simulink model "code_gen_man_bin"  (Simulink 7.5)
settings: Solver=FixedStepDiscrete  SolverMode=SingleTasking  StartTime=0.0  StopTime=10.0  FixedStep=0.01  RelTol=1e-3
InitFcn:
  | boat_constants
values from neighbouring files (symbols this model uses):
  figure8_waypoints = int32([ ... (first row only)    [boat_constants.m]
  InitialPoint = 0    [boat_constants.m]    (also in l2plus.m)
  IPStar = 0    [boat_constants.m]    (also in l2plus.m)
  ISA_g = 9.815    [boat_constants.m]
  MaxDwnPthStar = 1    [boat_constants.m]    (also in l2plus.m)
  OC2max = 49999    [boat_constants.m]    (also in simulation_constants.m)
  sampling_waypoints = int32([ ... (first row only)    [boat_constants.m]
  switchDistance = 4    [boat_constants.m]    (also in l2plus.m)
  T_step = 0.01    [boat_constants.m]    (also in common.m)
  tanIntercept = tan( 45*pi/180 )    [boat_constants.m]    (also in l2plus.m)
  test_waypoints = int32([ ... (first row only)    [boat_constants.m]
  TStar = single(4.5)    [boat_constants.m]    (also in l2plus.m = single(2))
  Turn2Track = 0    [boat_constants.m]    (also in l2plus.m)
  wheelbase = 3.27    [boat_constants.m]
undefined symbols (not defined in the file or in its folder): clearGpsData, clearSensorData, cpInitCommunications, DataEEInitAndClear, DataEEWrite, DiscIntNeverNeededParam, ecan1_buffered_transmit_matlab, ecan1_error_status_matlab, ecan1_init, GetAirData, getGpsData, getRevoData, getSensorData, GetThrottleData, GetWaterData, GetWindData, Init_onlyOnce, Init_Reset, initCalibrationRange, initGps, processNewCommData, processNewGpsData, processNewRevoData, setHilMode, u1, u2, uart1EnqueueStateData, uart2EnqueueActuatorData, y1
libraries: simulink x80, dsPICdrivers x50, uSimLib x4, simulink_need_slupdate x4
(part 4 of 6)

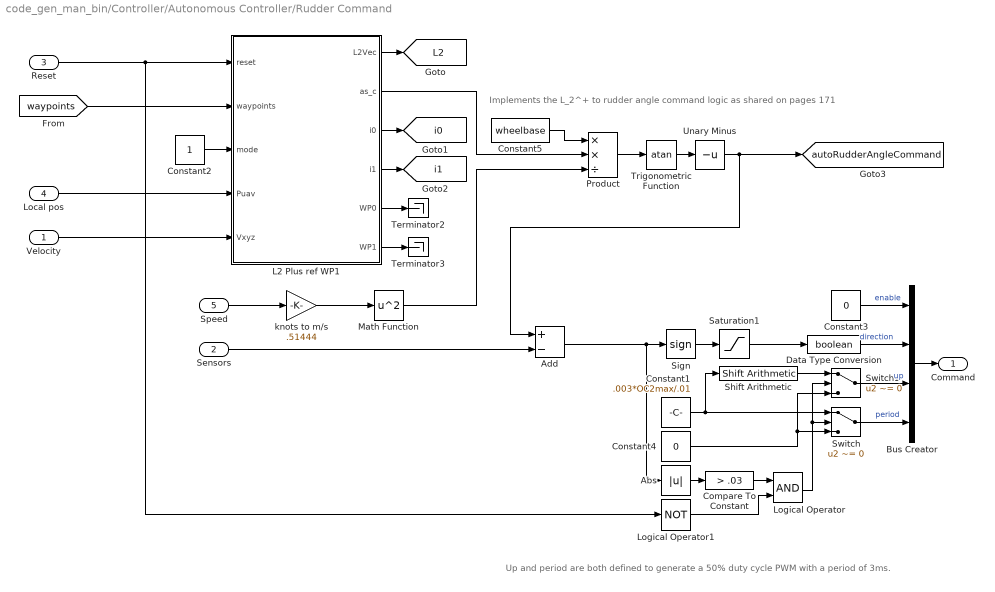
== system code_gen_man_bin/Controller/Autonomous Controller/Rudder Command ==
  note: Implements the L_2^+ to rudder angle command logic as shared on pages 171
  note: Up and period are both defined to generate a 50% duty cycle PWM with
      | a period of 3ms.
  Velocity : Inport
  Sensors : Inport  Port=2
  Reset : Inport  Port=3
  Local pos : Inport  Port=4
  Speed : Inport  Port=5
  Abs : Abs  OutDataType=fixdt(1, 16)  OutScaling=2^0
  Add : Sum  Inputs=+-  OutDataType=fixdt(1, 16)  OutScaling=2^-10
  Bus Creator : BusCreator
  Compare To Constant : simulink/Logic and Bit Operations/Compare To Constant  SystemSampleTime=-1  relop=>  const=.03  LogicOutDataTypeMode=boolean
  Constant1 : Constant  Value=.003*OC2max/.01  OutDataTypeMode=uint16  OutDataType=sfix(16)  OutScaling=2^0  OutDataTypeStr=uint16
  Constant2 : Constant  OutDataTypeMode=uint8  OutDataType=sfix(16)  OutScaling=2^0  OutDataTypeStr=uint8
  Constant3 : Constant  Value=0  OutDataTypeMode=boolean  OutDataType=sfix(16)  OutScaling=2^0  OutDataTypeStr=boolean
  Constant4 : Constant  Value=0  OutDataTypeMode=uint16  OutDataType=sfix(16)  OutScaling=2^0  OutDataTypeStr=uint16
  Constant5 : Constant  Value=wheelbase  OutDataTypeMode=boolean  OutDataType=sfix(16)  OutScaling=2^0  OutDataTypeStr=boolean
  Data Type Conversion : DataTypeConversion  OutDataTypeMode=boolean  OutDataType=fixdt(1, 16)  OutScaling=2^0  OutDataTypeStr=boolean  RndMeth=Simplest
  L2 Plus ref WP1 : Stateflow chart  TreatAsAtomicUnit=on
  Logical Operator : Logic  AllPortsSameDT=off  OutDataTypeMode=boolean  LogicDataType=fixdt(0, 8)  OutDataTypeStr=boolean
  Logical Operator1 : Logic  Operator=NOT  Inputs=1  AllPortsSameDT=off  OutDataTypeMode=boolean  LogicDataType=fixdt(0, 8)  OutDataTypeStr=boolean
  Math Function : Math  Operator=square  OutDataType=fixdt(1, 16)  OutScaling=2^0  SaturateOnIntegerOverflow=on
  Product : Product  Inputs=**/  OutDataType=fixdt(1, 16)  OutScaling=2^0  RndMeth=Zero
  Saturation1 : Saturate  UpperLimit=1  LowerLimit=0  OutDataTypeStr=Inherit: Inherit via back propagation
  Shift Arithmetic : simulink/Logic and Bit Operations/Shift Arithmetic  SystemSampleTime=-1  nBitShiftRight=1  nBinPtShiftRight=0
  Sign : Signum
  Switch : Switch  Criteria=u2 ~= 0  OutDataType=fixdt(1, 16)  OutScaling=2^0
  Switch1 : Switch  Criteria=u2 ~= 0  OutDataType=fixdt(1, 16)  OutScaling=2^0
  Terminator2 : Terminator
  Terminator3 : Terminator
  Trigonometric Function : Trigonometry  Operator=atan
  Unary Minus : UnaryMinus
  knots to m/s : Gain  Gain=.51444  ParameterDataType=fixdt(1, 16)  ParameterScaling=2^0  OutDataType=fixdt(1, 16)  OutScaling=2^0
  Command : Outport
  tag scope: L2=global, autoRudderAngleCommand=global, i0=global, i1=global
  wires:
  Unary Minus/1 -> [autoRudderAngleCommand], Add/1
  knots to m/s/1 -> Math Function/1
  Trigonometric Function/1 -> Unary Minus/1
  Product/1 -> Trigonometric Function/1
  Math Function/1 -> Product/3
  Constant5/1 -> Product/1
  L2 Plus ref WP1/6(WP1) -> Terminator3/1
  L2 Plus ref WP1/5(WP0) -> Terminator2/1
  L2 Plus ref WP1/2(as_c) -> Product/2
  Data Type Conversion/1 -> Bus Creator/2  "direction"
  Sensors/1 -> Add/2
  Bus Creator/1 -> Command/1
  Saturation1/1 -> Data Type Conversion/1
  Sign/1 -> Saturation1/1
  Constant2/1 -> L2 Plus ref WP1/3(mode)
  L2 Plus ref WP1/1(L2Vec) -> [L2]
  Velocity/1 -> L2 Plus ref WP1/5(Vxyz)
  Constant3/1 -> Bus Creator/1  "enable"
  Constant1/1 -> Shift Arithmetic/1, Switch/1
  Abs/1 -> Compare To Constant/1
  Shift Arithmetic/1 -> Switch1/1
  Switch/1 -> Bus Creator/4  "period"
  Switch1/1 -> Bus Creator/3  "up"
  Constant4/1 -> Switch/3, Switch1/3
  Reset/1 -> L2 Plus ref WP1/1(reset), Logical Operator1/1
  Local pos/1 -> L2 Plus ref WP1/4(Puav)
  L2 Plus ref WP1/3(i0) -> [i0]
  L2 Plus ref WP1/4(i1) -> [i1]
  Compare To Constant/1 -> Logical Operator/1
  Logical Operator/1 -> Switch/2, Switch1/2
  Logical Operator1/1 -> Logical Operator/2
  [waypoints] -> L2 Plus ref WP1/2(waypoints)
  Speed/1 -> knots to m/s/1
  Add/1 -> Sign/1, Abs/1

== system code_gen_man_bin/Controller/Autonomous Controller/State Keeper & Estimator ==
  throttle : Inport
  rudder : Inport  Port=2
  reset : Inport  Port=3
  gps : Inport  Port=4
  ballast : Inport  Port=5
  Ballast Estimator : Subsystem
  GPS Estimator : Subsystem
  Rudder Estimator : Subsystem
  Throttle Estimator : Subsystem
  sensors_t : Outport
  sensors_r : Outport  Port=2
  sensors_b : Outport  Port=3
  velocity : Outport  Port=4
  pos : Outport  Port=5
  heading : Outport  Port=6
  lla : Outport  Port=7
  datetime : Outport  Port=8
  tag scope: SensedGlobalPosition=global, SensedHeading=global, SensedLocalPosition=global, SensedVelocity=global
  wires:
  rudder/1 -> Rudder Estimator/1(r)
  ballast/1 -> Ballast Estimator/1(b)
  throttle/1 -> Throttle Estimator/1(t)
  reset/1 -> GPS Estimator/2(reset)
  GPS Estimator/1(velocity) -> velocity/1, [SensedVelocity]
  gps/1 -> GPS Estimator/1(gps)
  GPS Estimator/2(pos) -> pos/1, [SensedLocalPosition]
  GPS Estimator/3(heading) -> heading/1, [SensedHeading]
  GPS Estimator/4(lla) -> [SensedGlobalPosition], lla/1
  GPS Estimator/5(datetime) -> datetime/1
  Rudder Estimator/1(sensors_r) -> sensors_r/1
  Ballast Estimator/1(sensors_b) -> sensors_b/1
  Throttle Estimator/1(sensors_t) -> sensors_t/1

== system code_gen_man_bin/Controller/Autonomous Controller/Throttle Command ==
  sensors : Inport
  reset : Inport  Port=2
  Bus Creator : BusCreator
  Constant1 : Constant  Value=0  OutDataTypeMode=int16  OutDataType=sfix(16)  OutScaling=2^0  OutDataTypeStr=int16
  Constant5 : Constant  Value=1000  OutDataTypeMode=int16  OutDataType=sfix(16)  OutScaling=2^0  OutDataTypeStr=int16
  Mux Everything : Subsystem
  Switch : Switch  Criteria=u2 > Threshold  OutDataType=fixdt(1, 16)  OutScaling=2^0
  Terminator : Terminator
  Trigger Events : Subsystem
  command : Outport  OutDataType=sfix(16)  OutScaling=2^0
  tag scope: autoThrottleCommand=global
  wires:
  sensors/1 -> Terminator/1
  Bus Creator/1 -> command/1
  Trigger Events/1(Change Speed) -> Mux Everything/1(speed)
  Trigger Events/3(Enable) -> Mux Everything/3(enable)
  Trigger Events/2(Disable) -> Mux Everything/2(disable)
  reset/1 -> Trigger Events/2(Reset), Switch/2
  Mux Everything/1(iden) -> Bus Creator/1  "identifier"
  Mux Everything/2(data) -> Bus Creator/2  "data"
  Mux Everything/3(size) -> Bus Creator/3  "size"
  Mux Everything/4(trig) -> Bus Creator/4  "trigger"
  Switch/1 -> [autoThrottleCommand], Mux Everything/4(Throttle), Trigger Events/1(RC Throttle)
  Constant1/1 -> Switch/1
  Constant5/1 -> Switch/3

== system code_gen_man_bin/Controller/RC Inputs/Map PWM values to Actuator Signals ==
  rCmd : Inport
  tCmd : Inport  Port=2
  rAngle : Inport  Port=3
  Enable : EnablePort
  Manual Rudder Command : Subsystem
  Throttle Command : Subsystem
  Out1 : Outport
  Out2 : Outport  Port=2
  wires:
  rCmd/1 -> Manual Rudder Command/1(RC Rudder)
  Manual Rudder Command/1(Rudder Command) -> Out1/1
  tCmd/1 -> Throttle Command/1(speed)
  Throttle Command/1(command) -> Out2/1
  rAngle/1 -> Manual Rudder Command/2(rudderAngle)

== system code_gen_man_bin/Controller/Radio Control Inputs1/Calibration ==
  r : Inport  OutDataType=fixdt(1, 16)  OutScaling=2^0
  tr : Inport  Port=2  OutDataType=fixdt(1, 16)  OutScaling=2^0
  t : Inport  Port=3  OutDataType=fixdt(1, 16)  OutScaling=2^0
  Enable : EnablePort
  Data Store Read : DataStoreRead  DataStoreName=throttleRange  SampleTime=T_step
  Data Store Read1 : DataStoreRead  DataStoreName=rudderRange  SampleTime=T_step
  Data Store Read2 : DataStoreRead  DataStoreName=trackRange  SampleTime=T_step
  Data Store Write : DataStoreWrite  DataStoreName=throttleRange  SampleTime=-1
  Data Store Write1 : DataStoreWrite  DataStoreName=rudderRange  SampleTime=-1
  Data Store Write2 : DataStoreWrite  DataStoreName=trackRange  SampleTime=-1
  Data Type Conversion : DataTypeConversion  OutDataTypeMode=uint16  OutDataType=fixdt(1, 16)  OutScaling=2^0  OutDataTypeStr=uint16
  Data Type Conversion1 : DataTypeConversion  OutDataTypeMode=uint16  OutDataType=fixdt(1, 16)  OutScaling=2^0  OutDataTypeStr=uint16
  Data Type Conversion2 : DataTypeConversion  OutDataTypeMode=uint16  OutDataType=fixdt(1, 16)  OutScaling=2^0  OutDataTypeStr=uint16
  Store rudder range to memory : Subsystem
  Store throttle range to memory : Subsystem
  Store track range to memory : Subsystem
  Update range from input : Subsystem
  Update range from input1 : Subsystem
  Update range from input2 : Subsystem
  wires:
  Update range from input/1(newRange) -> Data Store Write1/1, Data Type Conversion/1
  Data Store Read1/1 -> Update range from input/1(limitRange)
  r/1 -> Update range from input/2(newValue)
  Update range from input2/1(newRange) -> Data Store Write2/1, Data Type Conversion2/1
  Data Store Read2/1 -> Update range from input2/1(limitRange)
  tr/1 -> Update range from input2/2(newValue)
  Update range from input1/1(newRange) -> Data Store Write/1, Data Type Conversion1/1
  Data Store Read/1 -> Update range from input1/1(limitRange)
  t/1 -> Update range from input1/2(newValue)
  Data Type Conversion/1 -> Store rudder range to memory/1(rudderRange)
  Data Type Conversion1/1 -> Store throttle range to memory/1(throttleRange)
  Data Type Conversion2/1 -> Store track range to memory/1(trackRange)

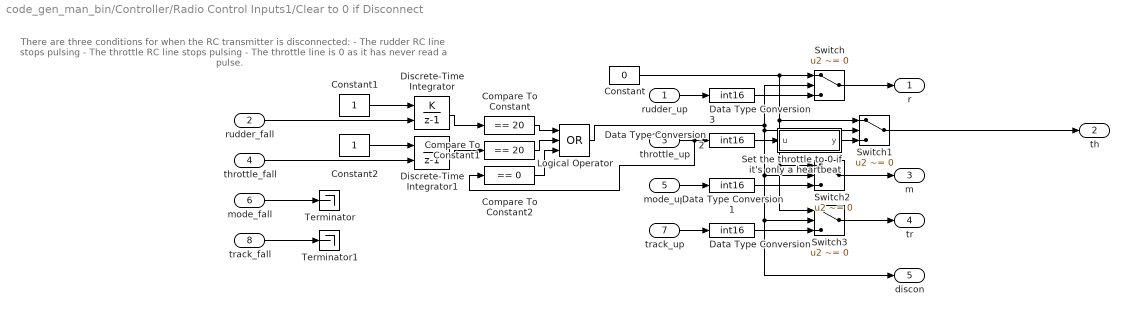
== system code_gen_man_bin/Controller/Radio Control Inputs1/Clear to 0 if Disconnect ==
  note: There are three conditions for when the RC transmitter is disconnected:
      |  - The rudder RC line stops pulsing
      |  - The throttle RC line stops pulsing
      |  - The throttle line is 0 as it has never read a pulse.
  rudder_up : Inport  OutDataType=sfix(16)  OutScaling=2^0
  rudder_fall : Inport  Port=2  OutDataType=sfix(16)  OutScaling=2^0
  throttle_up : Inport  Port=3  OutDataType=sfix(16)  OutScaling=2^0
  throttle_fall : Inport  Port=4  OutDataType=sfix(16)  OutScaling=2^0
  mode_up : Inport  Port=5  OutDataType=sfix(16)  OutScaling=2^0
  mode_fall : Inport  Port=6  OutDataType=sfix(16)  OutScaling=2^0
  track_up : Inport  Port=7  OutDataType=sfix(16)  OutScaling=2^0
  track_fall : Inport  Port=8  OutDataType=sfix(16)  OutScaling=2^0
  Compare To Constant : simulink/Logic and Bit Operations/Compare To Constant  SystemSampleTime=-1  relop===  const=20  LogicOutDataTypeMode=boolean
  Compare To Constant1 : simulink/Logic and Bit Operations/Compare To Constant  SystemSampleTime=-1  relop===  const=20  LogicOutDataTypeMode=boolean
  Compare To Constant2 : simulink/Logic and Bit Operations/Compare To Constant  SystemSampleTime=-1  relop===  const=0  LogicOutDataTypeMode=boolean
  Constant : Constant  Value=0  OutDataTypeMode=int16  OutDataType=sfix(16)  OutScaling=2^0  OutDataTypeStr=int16
  Constant1 : Constant  OutDataTypeMode=uint8  OutDataType=fixdt(1, 16)  OutScaling=2^0  OutDataTypeStr=uint8
  Constant2 : Constant  OutDataTypeMode=uint8  OutDataType=fixdt(1, 16)  OutScaling=2^0  OutDataTypeStr=uint8
  Data Type Conversion{,1..3} (4 alike) : DataTypeConversion  OutDataTypeMode=int16  OutDataType=fixdt(1, 16)  OutScaling=2^0  OutDataTypeStr=int16
  Discrete-Time Integrator : DiscreteIntegrator  IntegratorMethod=Accumulation: Forward Euler  ExternalReset=level  SampleTime=-1  OutDataType=fixdt(1, 16)  OutScaling=2^0  LimitOutput=on  UpperSaturationLimit=20  LowerSaturationLimit=0  ICPrevOutput=DiscIntNeverNeededParam  ICPrevScaledInput=DiscIntNeverNeededParam
  Discrete-Time Integrator1 : DiscreteIntegrator  IntegratorMethod=Accumulation: Forward Euler  ExternalReset=level  SampleTime=-1  OutDataType=fixdt(1, 16)  OutScaling=2^0  LimitOutput=on  UpperSaturationLimit=20  LowerSaturationLimit=0  ICPrevOutput=DiscIntNeverNeededParam  ICPrevScaledInput=DiscIntNeverNeededParam
  Logical Operator : Logic  Operator=OR  Inputs=3  AllPortsSameDT=off  OutDataTypeMode=boolean  LogicDataType=fixdt(0, 8)  OutDataTypeStr=boolean
  Set the throttle to 0 if it's only a heartbeat : Stateflow chart  TreatAsAtomicUnit=on
  Switch{,1..3} (4 alike) : Switch  Criteria=u2 ~= 0  Threshold=40
  Terminator : Terminator
  Terminator1 : Terminator
  r : Outport  OutDataType=sfix(16)  OutScaling=2^0
  th : Outport  Port=2  OutDataType=sfix(16)  OutScaling=2^0
  m : Outport  Port=3  OutDataType=sfix(16)  OutScaling=2^0
  tr : Outport  Port=4  OutDataType=sfix(16)  OutScaling=2^0
  discon : Outport  Port=5  OutDataType=sfix(16)  OutScaling=2^0
  wires:
  Switch1/1 -> th/1
  throttle_up/1 -> Data Type Conversion2/1, Compare To Constant2/1
  Switch/1 -> r/1
  rudder_up/1 -> Data Type Conversion3/1
  Constant/1 -> Switch/1, Switch1/1, Switch2/1, Switch3/1
  Switch2/1 -> m/1
  mode_up/1 -> Data Type Conversion1/1
  track_up/1 -> Data Type Conversion/1
  Switch3/1 -> tr/1
  rudder_fall/1 -> Discrete-Time Integrator/2
  mode_fall/1 -> Terminator/1
  track_fall/1 -> Terminator1/1
  Constant1/1 -> Discrete-Time Integrator/1
  throttle_fall/1 -> Discrete-Time Integrator1/2
  Data Type Conversion/1 -> Switch3/3
  Data Type Conversion1/1 -> Switch2/3
  Data Type Conversion2/1 -> Set the throttle to 0 if it's only a heartbeat/1(u)
  Data Type Conversion3/1 -> Switch/3
  Constant2/1 -> Discrete-Time Integrator1/1
  Logical Operator/1 -> Switch/2, Switch1/2, Switch2/2, Switch3/2, discon/1
  Discrete-Time Integrator1/1 -> Compare To Constant1/1
  Discrete-Time Integrator/1 -> Compare To Constant/1
  Compare To Constant/1 -> Logical Operator/1
  Compare To Constant1/1 -> Logical Operator/2
  Compare To Constant2/1 -> Logical Operator/3
  Set the throttle to 0 if it's only a heartbeat/1(y) -> Switch1/3

== system code_gen_man_bin/Controller/Radio Control Inputs1/Detect calibration trigger ==
  note: This part checks for a mode change and checks that
      | it isn't the result of a disconnect. We don't want those
      | to accidently trigger a calibration.
  mode : Inport
  value : Inport  Port=2
  Calibration mode (LED D6) : dsPICdrivers/Digital I//O/Digital Output Write  Tag=dsPIC_Digital_Output  Priority=5  PORT=A  Pin=3  Simultaneous=off  OrderingInOutPopup=None
  Compare To Constant1 : simulink/Logic and Bit Operations/Compare To Constant  SystemSampleTime=-1  relop=>  const=0  LogicOutDataTypeMode=uint8
  Compute Calibration State : Stateflow chart  TreatAsAtomicUnit=on
  Data Store Memory : DataStoreMemory  DataStoreName=restoredCalibration  ReadBeforeWriteMsg=warning  WriteAfterWriteMsg=warning  WriteAfterReadMsg=warning  DataType=boolean  OutDataType=fixdt(1, 16)  OutScaling=2^0  OutDataTypeStr=boolean
      settings: RTWStateStorageClass=ExportedGlobal
  Data Store Read1 : DataStoreRead  DataStoreName=restoredCalibration  SampleTime=T_step
  Detect Change1 : simulink/Logic and Bit Operations/Detect Change  SystemSampleTime=-1  vinit=0
  Logical Operator : Logic  AllPortsSameDT=off  OutDataTypeMode=boolean  LogicDataType=fixdt(0, 8)  OutDataTypeStr=boolean
  State outputs : Subsystem
  calibrateState : Outport  OutDataType=fixdt(1, 16)  OutScaling=2^0
  wires:
  mode/1 -> Detect Change1/1
  Logical Operator/1 -> Compute Calibration State/1(trigger)
  State outputs/1(LED) -> Calibration mode (LED D6)/1
  value/1 -> Compare To Constant1/1
  Detect Change1/1 -> Logical Operator/1
  Compare To Constant1/1 -> Logical Operator/2
  Compute Calibration State/1(state) -> calibrateState/1, State outputs/1(cState)
  Data Store Read1/1 -> Compute Calibration State/2(restoredCalibration)

== system code_gen_man_bin/Controller/Radio Control Inputs1/If Action Subsystem ==
  Action Port : ActionPort  ActionType=then
  Constant : Constant  Value=0  OutDataTypeMode=single  OutDataType=fixdt(1, 16)  OutScaling=2^0  OutDataTypeStr=single
  Out1 : Outport  OutDataType=fixdt(1, 16)  OutScaling=2^0  InitialOutput=50
  wires:
  Constant/1 -> Out1/1

== system code_gen_man_bin/Controller/Radio Control Inputs1/If Action Subsystem1 ==
  note: This subsystem maps the input RC range into tenths of a degree and then
      | outputs the result as a float in units of radians. It follows the convention where
      | positive angles are to port and negative angles are to starboard.
  input : Inport  OutDataType=fixdt(1, 16)  OutScaling=2^0
  range : Inport  Port=2  OutDataType=fixdt(1, 16)  OutScaling=2^0
  Action Port : ActionPort  ActionType=else
  Add 8% center deadband : Subsystem
  Add binning : Stateflow chart  TreatAsAtomicUnit=on
  Constant : Constant  Value=-450  OutDataType=fixdt(1, 16)  OutScaling=2^0  OutDataTypeStr=Inherit: Inherit via back propagation
  Constant1 : Constant  Value=450  OutDataType=fixdt(1, 16)  OutScaling=2^0  OutDataTypeStr=Inherit: Inherit via back propagation
  Data Type Conversion : DataTypeConversion  OutDataType=fixdt(1, 16)  OutScaling=2^0
  Data Type Conversion1 : DataTypeConversion  OutDataType=fixdt(1, 16)  OutScaling=2^0
  Data Type Conversion2 : DataTypeConversion  OutDataTypeMode=single  OutDataType=fixdt(1, 16)  OutScaling=2^0  OutDataTypeStr=single
  Demux : Demux  Outputs=2
  Gain : Gain  Gain=pi/1800  ParameterDataType=fixdt(1, 16)  ParameterScaling=2^0  OutDataType=fixdt(1, 16)  OutScaling=2^0
  Map into range : Stateflow chart  TreatAsAtomicUnit=on
  Saturation : Saturate  UpperLimit=450  LowerLimit=-450  OutDataTypeMode=int16  OutDataType=fixdt(1, 16)  OutScaling=2^0  OutDataTypeStr=int16  RndMeth=Simplest
  Weighted Moving Average : simulink_need_slupdate/Weighted Moving Average  mgainval=[.1 .1 .1 .1 .1 .1 .1 .1 .1 .1]  vinit=0.0  samptime=-1  OutDataTypeStr=Inherit: Inherit via back propagation  OutDataType=sfix(16)  OutScaling=2^-10  DoSatur=off  GainDataType=uint(16)  MatRadixGroup=Best Precision: Matrix-wise  GainScaling=2^-10
  Out1 : Outport  OutDataType=fixdt(1, 16)  OutScaling=2^0  InitialOutput=50
  wires:
  Constant1/1 -> Map into range/5(out_max)
  Constant/1 -> Map into range/4(out_min)
  Demux/1 -> Map into range/2(in_min)
  Demux/2 -> Map into range/3(in_max)
  range/1 -> Data Type Conversion1/1
  Map into range/1(mappedValue) -> Saturation/1
  Data Type Conversion/1 -> Map into range/1(val)
  Data Type Conversion1/1 -> Demux/1
  input/1 -> Data Type Conversion/1
  Add 8% center deadband/1(Out1) -> Weighted Moving Average/1
  Saturation/1 -> Add 8% center deadband/1(In1)
  Gain/1 -> Add binning/1(manualRudderAngle)
  Data Type Conversion2/1 -> Gain/1
  Weighted Moving Average/1 -> Data Type Conversion2/1
  Add binning/1(newManualRudderAngle) -> Out1/1

== system code_gen_man_bin/Controller/Radio Control Inputs1/If Action Subsystem2 ==
  Action Port : ActionPort  ActionType=then
  Constant : Constant  Value=0  OutDataType=fixdt(1, 16)  OutScaling=2^0  OutDataTypeStr=Inherit: Inherit via back propagation
  Out1 : Outport  OutDataType=fixdt(1, 16)  OutScaling=2^0  InitialOutput=0
  wires:
  Constant/1 -> Out1/1

== system code_gen_man_bin/Controller/Radio Control Inputs1/If Action Subsystem3 ==
  input : Inport  OutDataType=fixdt(1, 16)  OutScaling=2^0
  range : Inport  Port=2  OutDataType=fixdt(1, 16)  OutScaling=2^0
  Action Port : ActionPort  ActionType=else
  Add 5% deadband about 0 : Subsystem
  Constant : Constant  Value=-700  OutDataType=fixdt(1, 16)  OutScaling=2^0  OutDataTypeStr=Inherit: Inherit via back propagation
  Constant1 : Constant  Value=1000  OutDataType=fixdt(1, 16)  OutScaling=2^0  OutDataTypeStr=Inherit: Inherit via back propagation
  Data Type Conversion : DataTypeConversion  OutDataType=fixdt(1, 16)  OutScaling=2^0
  Data Type Conversion1 : DataTypeConversion  OutDataType=fixdt(1, 16)  OutScaling=2^0
  Demux : Demux  Outputs=2
  Map into range : Stateflow chart  TreatAsAtomicUnit=on
  Saturation : Saturate  UpperLimit=1000  LowerLimit=-700  OutDataTypeMode=int16  OutDataType=fixdt(1, 16)  OutScaling=2^0  OutDataTypeStr=int16  RndMeth=Simplest
  Out1 : Outport  OutDataType=fixdt(1, 16)  OutScaling=2^0  InitialOutput=0
  wires:
  Constant1/1 -> Map into range/5(out_max)
  Constant/1 -> Map into range/4(out_min)
  Demux/1 -> Map into range/2(in_min)
  Demux/2 -> Map into range/3(in_max)
  range/1 -> Data Type Conversion1/1
  Map into range/1(mappedValue) -> Saturation/1
  Data Type Conversion/1 -> Map into range/1(val)
  Data Type Conversion1/1 -> Demux/1
  Saturation/1 -> Add 5% deadband about 0/1(In1)
  input/1 -> Data Type Conversion/1
  Add 5% deadband about 0/1(Out1) -> Out1/1

== system code_gen_man_bin/Controller/Radio Control Inputs1/If Action Subsystem4 ==
  Action Port : ActionPort  ActionType=then
  Constant : Constant  Value=500  OutDataType=fixdt(1, 16)  OutScaling=2^0  OutDataTypeStr=Inherit: Inherit via back propagation
  Out1 : Outport  OutDataType=fixdt(1, 16)  OutScaling=2^0  InitialOutput=50
  wires:
  Constant/1 -> Out1/1

== system code_gen_man_bin/Controller/Radio Control Inputs1/If Action Subsystem5 ==
  input : Inport  OutDataType=fixdt(1, 16)  OutScaling=2^0
  range : Inport  Port=2  OutDataType=fixdt(1, 16)  OutScaling=2^0
  Action Port : ActionPort  ActionType=else
  Add 8% center deadband : Subsystem
  Constant : Constant  Value=0  OutDataType=fixdt(1, 16)  OutScaling=2^0  OutDataTypeStr=Inherit: Inherit via back propagation
  Constant1 : Constant  Value=1000  OutDataType=fixdt(1, 16)  OutScaling=2^0  OutDataTypeStr=Inherit: Inherit via back propagation
  Data Type Conversion : DataTypeConversion  OutDataType=fixdt(1, 16)  OutScaling=2^0
  Data Type Conversion1 : DataTypeConversion  OutDataType=fixdt(1, 16)  OutScaling=2^0
  Demux : Demux  Outputs=2
  Map into range : Stateflow chart  TreatAsAtomicUnit=on
  Saturation : Saturate  UpperLimit=1000  LowerLimit=0  OutDataTypeMode=int16  OutDataType=fixdt(1, 16)  OutScaling=2^0  OutDataTypeStr=int16  RndMeth=Simplest
  Out1 : Outport  OutDataType=fixdt(1, 16)  OutScaling=2^0  InitialOutput=50
  wires:
  Constant1/1 -> Map into range/5(out_max)
  Constant/1 -> Map into range/4(out_min)
  Demux/1 -> Map into range/2(in_min)
  Demux/2 -> Map into range/3(in_max)
  range/1 -> Data Type Conversion1/1
  Map into range/1(mappedValue) -> Saturation/1
  Data Type Conversion/1 -> Map into range/1(val)
  Data Type Conversion1/1 -> Demux/1
  Saturation/1 -> Add 8% center deadband/1(In1)
  input/1 -> Data Type Conversion/1
  Add 8% center deadband/1(Out1) -> Out1/1

== system code_gen_man_bin/Controller/Radio Control Inputs1/Reset calibration range ==
  note: Reset the calibration range for each
      | channel before recalibration.
  Trigger : TriggerPort
  Constant1 : Constant  Value=[8000 8000]  OutDataType=fixdt(1, 16)  OutScaling=2^0  OutDataTypeStr=Inherit: Inherit via back propagation  SampleTime=Inf
  Data Store Write : DataStoreWrite  DataStoreName=throttleRange  SampleTime=-1
  Data Store Write1 : DataStoreWrite  DataStoreName=rudderRange  SampleTime=-1
  Data Store Write2 : DataStoreWrite  DataStoreName=trackRange  SampleTime=-1
  wires:
  Constant1/1 -> Data Store Write/1, Data Store Write1/1, Data Store Write2/1

== system code_gen_man_bin/Controller/Rudder sensor calibration/Rudder Command ==
  note: Up and period are both defined to generate a 50% duty cycle PWM with
      | a period of 3ms.
  step : Inport
  dir : Inport  Port=2
  Bus Creator : BusCreator
  Constant1 : Constant  Value=.003*OC2max/.01  OutDataTypeMode=uint16  OutDataType=sfix(16)  OutScaling=2^0  OutDataTypeStr=uint16
  Constant3 : Constant  Value=0  OutDataTypeMode=boolean  OutDataType=sfix(16)  OutScaling=2^0  OutDataTypeStr=boolean
  Constant4 : Constant  Value=0  OutDataTypeMode=uint16  OutDataType=sfix(16)  OutScaling=2^0  OutDataTypeStr=uint16
  Shift Arithmetic : simulink/Logic and Bit Operations/Shift Arithmetic  SystemSampleTime=-1  nBitShiftRight=1  nBinPtShiftRight=0
  Switch : Switch  Criteria=u2 ~= 0  OutDataType=fixdt(1, 16)  OutScaling=2^0
  Switch1 : Switch  Criteria=u2 ~= 0  OutDataType=fixdt(1, 16)  OutScaling=2^0
  Command : Outport
  wires:
  step/1 -> Switch1/2, Switch/2
  Constant4/1 -> Switch1/3, Switch/3
  Switch1/1 -> Bus Creator/3  "up"
  Switch/1 -> Bus Creator/4  "period"
  Shift Arithmetic/1 -> Switch1/1
  Constant1/1 -> Switch/1, Shift Arithmetic/1
  Constant3/1 -> Bus Creator/1  "enable"
  Bus Creator/1 -> Command/1
  dir/1 -> Bus Creator/2  "direction"

== system code_gen_man_bin/Controller/Rudder sensor calibration/Throttle Command ==
  en : Inport
  Bus Creator : BusCreator
  Logical Operator : Logic  Operator=NOT  AllPortsSameDT=off  OutDataTypeMode=boolean  LogicDataType=fixdt(0, 8)  OutDataTypeStr=boolean
  Mux Everything : Subsystem
  command : Outport  OutDataType=sfix(16)  OutScaling=2^0
  wires:
  Mux Everything/3(size) -> Bus Creator/3  "size"
  Mux Everything/2(data) -> Bus Creator/2  "data"
  Mux Everything/1(iden) -> Bus Creator/1  "identifier"
  en/1 -> Logical Operator/1
  Bus Creator/1 -> command/1
  Logical Operator/1 -> Mux Everything/1(reset)
  Mux Everything/4(trig) -> Bus Creator/4  "trigger"

== system code_gen_man_bin/Controller/Split trackCommand to singular commands/Countdown timer for trigger ==
  note: calibrationState is a uint8 with 3 states:
      | 0 is off,
      | 1 is timing down waiting to transition,
      | 2 is after a successful transition
  in : Inport
  Constant1 : Constant  OutDataTypeMode=uint8  OutDataType=fixdt(1, 16)  OutScaling=2^0  OutDataTypeStr=uint8  SampleTime=T_step
  Data Store Memory : DataStoreMemory  DataStoreName=timerState  ReadBeforeWriteMsg=warning  WriteAfterWriteMsg=warning  WriteAfterReadMsg=warning  DataType=uint8  OutDataType=fixdt(1, 16)  OutScaling=2^0  OutDataTypeStr=uint8
  Data Store Read : DataStoreRead  DataStoreName=timerState  SampleTime=T_step
  Data Type Conversion1 : DataTypeConversion  OutDataTypeMode=uint8  OutDataType=fixdt(1, 16)  OutScaling=2^0  OutDataTypeStr=uint8
  State transitions : Subsystem
  Timer : DiscreteIntegrator  gainval=100  ExternalReset=level  InitialConditionMode=State only (most efficient)  SampleTime=T_step  OutDataTypeMode=uint8  OutDataType=fixdt(1, 16)  OutScaling=2^0  OutDataTypeStr=uint8  RndMeth=Simplest  LimitOutput=on  UpperSaturationLimit=127  LowerSaturationLimit=0  ICPrevOutput=DiscIntNeverNeededParam  ICPrevScaledInput=DiscIntNeverNeededParam
  Unit Delay2 : UnitDelay  SampleTime=-1
  trigger : Outport  OutDataType=fixdt(1, 16)  OutScaling=2^0
  wires:
  Constant1/1 -> Timer/1
  Timer/1 -> State transitions/1(timer)
  Data Store Read/1 -> State transitions/3(timerState)
  Unit Delay2/1 -> Timer/2
  State transitions/1(startTimer) -> Unit Delay2/1
  in/1 -> Data Type Conversion1/1
  Data Type Conversion1/1 -> State transitions/2(level)
  State transitions/2(trigger) -> trigger/1

== system code_gen_man_bin/Controller/Split trackCommand to singular commands/Countdown timer for trigger1 ==
  note: calibrationState is a uint8 with 3 states:
      | 0 is off,
      | 1 is timing down waiting to transition,
      | 2 is after a successful transition
  in : Inport
  Constant1 : Constant  OutDataTypeMode=uint8  OutDataType=fixdt(1, 16)  OutScaling=2^0  OutDataTypeStr=uint8  SampleTime=T_step
  Data Store Memory : DataStoreMemory  DataStoreName=timerState2  ReadBeforeWriteMsg=warning  WriteAfterWriteMsg=warning  WriteAfterReadMsg=warning  DataType=uint8  OutDataType=fixdt(1, 16)  OutScaling=2^0  OutDataTypeStr=uint8
  Data Store Read : DataStoreRead  DataStoreName=timerState2  SampleTime=T_step
  Data Type Conversion1 : DataTypeConversion  OutDataTypeMode=uint8  OutDataType=fixdt(1, 16)  OutScaling=2^0  OutDataTypeStr=uint8
  State transitions : Subsystem
  Timer : DiscreteIntegrator  gainval=100  ExternalReset=level  InitialConditionMode=State only (most efficient)  SampleTime=T_step  OutDataTypeMode=uint8  OutDataType=fixdt(1, 16)  OutScaling=2^0  OutDataTypeStr=uint8  RndMeth=Simplest  LimitOutput=on  UpperSaturationLimit=127  LowerSaturationLimit=0  ICPrevOutput=DiscIntNeverNeededParam  ICPrevScaledInput=DiscIntNeverNeededParam
  Unit Delay2 : UnitDelay  SampleTime=-1
  trigger : Outport  OutDataType=fixdt(1, 16)  OutScaling=2^0
  wires:
  State transitions/2(trigger) -> trigger/1
  Data Type Conversion1/1 -> State transitions/2(level)
  in/1 -> Data Type Conversion1/1
  State transitions/1(startTimer) -> Unit Delay2/1
  Unit Delay2/1 -> Timer/2
  Data Store Read/1 -> State transitions/3(timerState)
  Timer/1 -> State transitions/1(timer)
  Constant1/1 -> Timer/1

== system code_gen_man_bin/Transmit actuator data/Package and Transmit Sensor Struct/Build HIL sentence ==
  data : Inport
  Bitwise Operator : simulink/Logic and Bit Operations/Bitwise Operator  logicop=XOR  UseBitMask=off  BitMask=bin2dec('11011001')  BitMaskRealWorld=Stored Integer
  Constant : Constant  Value=37  OutDataTypeMode=uint8  OutDataType=fixdt(1, 16)  OutScaling=2^0  OutDataTypeStr=uint8
  Constant1 : Constant  Value=38  OutDataTypeMode=uint8  OutDataType=fixdt(1, 16)  OutScaling=2^0  OutDataTypeStr=uint8
  Constant2 : Constant  Value=94  OutDataTypeMode=uint8  OutDataType=fixdt(1, 16)  OutScaling=2^0  OutDataTypeStr=uint8
  Constant3 : Constant  Value=38  OutDataTypeMode=uint8  OutDataType=fixdt(1, 16)  OutScaling=2^0  OutDataTypeStr=uint8
  Constant4 : Constant  Value=2  OutDataTypeMode=uint8  OutDataType=fixdt(1, 16)  OutScaling=2^0  OutDataTypeStr=uint8
  Mux2 : Mux  Inputs=3
  Pack : Stateflow chart  TreatAsAtomicUnit=on
  Probe : Probe  ProbeSampleTime=off  ProbeComplexSignal=off  ProbeWidthDataType=uint8
  sent : Outport
  wires:
  data/1 -> Probe/1, Mux2/3
  Constant/1 -> Pack/1(a)
  Constant1/1 -> Pack/2(b)
  Pack/1(y) -> sent/1
  Mux2/1 -> Bitwise Operator/1, Pack/3(c)
  Probe/1 -> Mux2/2
  Constant2/1 -> Pack/4(d)
  Constant3/1 -> Pack/5(e)
  Bitwise Operator/1 -> Pack/6(f)
  Constant4/1 -> Mux2/1

== system code_gen_man_bin/Controller/Autonomous Controller/State Keeper & Estimator/Ballast Estimator ==
  b : Inport
  Bus Selector1 : BusSelector  OutputSignals=position
  sensors_b : Outport
  wires:
  b/1 -> Bus Selector1/1
  Bus Selector1/1 -> sensors_b/1  "<position>"

== system code_gen_man_bin/Controller/Autonomous Controller/State Keeper & Estimator/GPS Estimator ==
  gps : Inport
  reset : Inport  Port=2  OutDataType=fixdt(1, 16)  OutScaling=2^0
  Add : Sum  OutDataType=fixdt(1, 16)  OutScaling=2^-10
  Bus Selector1 : BusSelector  OutputSignals=latitude,longitude,altitude,newData
  Calculate local position via velocity integral between true GPS updates : Stateflow chart  TreatAsAtomicUnit=on
  Discrete-Time Integrator4 : DiscreteIntegrator  ExternalReset=level  SampleTime=-1  OutDataType=fixdt(1, 16)  OutScaling=2^0  ICPrevOutput=DiscIntNeverNeededParam  ICPrevScaledInput=DiscIntNeverNeededParam
  Mux1 : Mux  Inputs=3
  Subsystem : Subsystem
  velocity : Outport
  pos : Outport  Port=2
  heading : Outport  Port=3
  lla : Outport  Port=4
  datetime : Outport  Port=5
  wires:
  reset/1 -> Calculate local position via velocity integral between true GPS updates/3(reset)
  Subsystem/2(heading) -> heading/1
  gps/1 -> Subsystem/1(gps), Bus Selector1/1
  Subsystem/3(pos) -> lla/1
  Subsystem/4(time) -> datetime/1
  Discrete-Time Integrator4/1 -> Add/2
  Add/1 -> pos/1
  Bus Selector1/1 -> Mux1/1  "<latitude>"
  Bus Selector1/2 -> Mux1/2  "<longitude>"
  Bus Selector1/3 -> Mux1/3  "<altitude>"
  Bus Selector1/4 -> Calculate local position via velocity integral between true GPS updates/2(newData)  "<newData>"
  Mux1/1 -> Calculate local position via velocity integral between true GPS updates/1(latLonAlt)
  Calculate local position via velocity integral between true GPS updates/2(resetIntegrator) -> Discrete-Time Integrator4/2
  Calculate local position via velocity integral between true GPS updates/1(localPosition) -> Add/1
  Subsystem/1(velocity) -> velocity/1, Discrete-Time Integrator4/1

== system code_gen_man_bin/Controller/Autonomous Controller/State Keeper & Estimator/Rudder Estimator ==
  r : Inport
  sensors_r : Outport
  wires:
  r/1 -> sensors_r/1

== system code_gen_man_bin/Controller/Autonomous Controller/State Keeper & Estimator/Throttle Estimator ==
  t : Inport
  sensors_t : Outport
  wires:
  t/1 -> sensors_t/1

== system code_gen_man_bin/Controller/Autonomous Controller/Throttle Command/Mux Everything ==
  speed : Inport  OutDataType=sfix(16)  OutScaling=2^0
  disable : Inport  Port=2  OutDataType=sfix(16)  OutScaling=2^0
  enable : Inport  Port=3  OutDataType=sfix(16)  OutScaling=2^0
  Throttle : Inport  Port=4  OutDataType=sfix(16)  OutScaling=2^0
  0x300 : Constant  Value=768  OutDataTypeMode=uint32  OutDataType=sfix(16)  OutScaling=2^0  OutDataTypeStr=uint32
  0x301 : Constant  Value=769  OutDataTypeMode=uint32  OutDataType=sfix(16)  OutScaling=2^0  OutDataTypeStr=uint32
  Build speed command : Subsystem
  Disable motor : Constant  Value=[0 0 0 0 64 0]  OutDataTypeMode=uint8  OutDataType=sfix(16)  OutScaling=2^0  OutDataTypeStr=uint8
  Enable motor : Constant  Value=[0 0 0 0 32 0]  OutDataTypeMode=uint8  OutDataType=sfix(16)  OutScaling=2^0  OutDataTypeStr=uint8
  Logical Operator1 : Logic  Operator=OR  AllPortsSameDT=off  OutDataTypeMode=boolean  OutDataTypeStr=boolean
  Message Length1 : Probe  ProbeSampleTime=off  ProbeComplexSignal=off  ProbeWidthDataType=uint8
  Multiport Switch : MultiPortSwitch  zeroidx=off
  Multiport Switch1 : MultiPortSwitch  zeroidx=off
  Select data packet : Stateflow chart  TreatAsAtomicUnit=on
  Switch : Switch  Criteria=u2 ~= 0
  iden : Outport  OutDataType=sfix(16)  OutScaling=2^0
  data : Outport  Port=2  OutDataType=sfix(16)  OutScaling=2^0
  size : Outport  Port=3  OutDataType=sfix(16)  OutScaling=2^0
  trig : Outport  Port=4  OutDataType=sfix(16)  OutScaling=2^0
  wires:
  Enable motor/1 -> Multiport Switch/3
  Disable motor/1 -> Multiport Switch/2
  Throttle/1 -> Build speed command/1(CC)
  Multiport Switch/1 -> Message Length1/1, data/1
  Message Length1/1 -> size/1
  0x300/1 -> Switch/1
  0x301/1 -> Switch/3
  Switch/1 -> iden/1
  disable/1 -> Logical Operator1/1, Select data packet/1(dis), Multiport Switch1/2
  enable/1 -> Logical Operator1/2, Select data packet/2(en), Multiport Switch1/3
  Logical Operator1/1 -> Switch/2
  Select data packet/1(y) -> Multiport Switch/1, Multiport Switch1/1
  Multiport Switch1/1 -> trig/1
  speed/1 -> Multiport Switch1/4
  Build speed command/1(msg) -> Multiport Switch/4

== system code_gen_man_bin/Controller/Autonomous Controller/Throttle Command/Trigger Events ==
  RC Throttle : Inport  OutDataType=sfix(16)  OutScaling=2^0
  Reset : Inport  Port=2  OutDataType=sfix(16)  OutScaling=2^0
  Data Type Conversion1 : DataTypeConversion  OutDataTypeMode=boolean  OutDataType=sfix(16)  OutScaling=2^0  OutDataTypeStr=boolean
  Data Type Conversion2 : DataTypeConversion  OutDataTypeMode=boolean  OutDataType=sfix(16)  OutScaling=2^0  OutDataTypeStr=boolean
  Data Type Conversion3 : DataTypeConversion  OutDataTypeMode=boolean  OutDataType=sfix(16)  OutScaling=2^0  OutDataTypeStr=boolean
  Detect Change : simulink/Logic and Bit Operations/Detect Change  SystemSampleTime=-1  vinit=0
  Detect Fall Nonpositive : simulink/Logic and Bit Operations/Detect Fall Nonpositive  SystemSampleTime=-1  vinit=0
  Detect Rise Positive : simulink/Logic and Bit Operations/Detect Rise Positive  SystemSampleTime=-1  vinit=0
  Shift Arithmetic : simulink/Logic and Bit Operations/Shift Arithmetic  SystemSampleTime=-1  nBitShiftRight=2  nBinPtShiftRight=0
  Weighted Moving Average : simulink_need_slupdate/Weighted Moving Average  mgainval=[.5 .5]  vinit=0.0  samptime=-1  OutDataTypeStr=Inherit: Inherit via back propagation  OutDataType=sfix(16)  OutScaling=2^-10  DoSatur=off  GainDataType=uint(16)  MatRadixGroup=Best Precision: Matrix-wise  GainScaling=2^-10
  Change Speed : Outport  OutDataType=sfix(16)  OutScaling=2^0
  Disable : Outport  Port=2  OutDataType=sfix(16)  OutScaling=2^0
  Enable : Outport  Port=3  OutDataType=sfix(16)  OutScaling=2^0
  wires:
  RC Throttle/1 -> Shift Arithmetic/1
  Detect Change/1 -> Data Type Conversion3/1
  Weighted Moving Average/1 -> Detect Change/1
  Shift Arithmetic/1 -> Weighted Moving Average/1
  Reset/1 -> Detect Fall Nonpositive/1, Detect Rise Positive/1
  Detect Fall Nonpositive/1 -> Data Type Conversion2/1
  Detect Rise Positive/1 -> Data Type Conversion1/1
  Data Type Conversion3/1 -> Change Speed/1
  Data Type Conversion2/1 -> Enable/1
  Data Type Conversion1/1 -> Disable/1

== system code_gen_man_bin/Controller/RC Inputs/Map PWM values to Actuator Signals/Manual Rudder Command ==
  note: This subsystem wraps the RC rudder command inside a proportional controller. It follows the same
      | logic used within the Autonomous Controller.
  note: Enable is an active-low signal for the 2035
      | driver board currently being used.
  RC Rudder : Inport  OutDataType=sfix(16)  OutScaling=2^0
  rudderAngle : Inport  Port=2  OutDataType=sfix(16)  OutScaling=2^0
  Abs : Abs  OutDataType=fixdt(1, 16)  OutScaling=2^0
  Add : Sum  Inputs=-+  OutDataType=fixdt(1, 16)  OutScaling=2^-10
  Bus Creator1 : BusCreator
  Compare To Constant : simulink/Logic and Bit Operations/Compare To Constant  SystemSampleTime=-1  relop=>  const=.03  LogicOutDataTypeMode=boolean
  Constant3 : Constant  Value=.003*OC2max/.01  OutDataTypeMode=uint16  OutDataType=sfix(16)  OutScaling=2^0  OutDataTypeStr=uint16
  Constant5 : Constant  Value=0  OutDataTypeMode=boolean  OutDataType=sfix(16)  OutScaling=2^0  OutDataTypeStr=boolean
  Constant6 : Constant  Value=0  OutDataTypeMode=uint16  OutDataType=sfix(16)  OutScaling=2^0  OutDataTypeStr=uint16
  Data Type Conversion : DataTypeConversion  OutDataTypeMode=boolean  OutDataType=fixdt(1, 16)  OutScaling=2^0  OutDataTypeStr=boolean  RndMeth=Simplest
  Saturation1 : Saturate  UpperLimit=1  LowerLimit=0  OutDataTypeStr=Inherit: Inherit via back propagation
  Shift Arithmetic1 : simulink/Logic and Bit Operations/Shift Arithmetic  SystemSampleTime=-1  nBitShiftRight=1  nBinPtShiftRight=0
  Sign : Signum
  Switch2 : Switch  Criteria=u2 ~= 0  OutDataType=fixdt(1, 16)  OutScaling=2^0
  Switch3 : Switch  Criteria=u2 ~= 0  OutDataType=fixdt(1, 16)  OutScaling=2^0
  Rudder Command : Outport
  wires:
  RC Rudder/1 -> Add/2
  Bus Creator1/1 -> Rudder Command/1
  Add/1 -> Abs/1, Sign/1
  Compare To Constant/1 -> Switch3/2, Switch2/2
  Constant6/1 -> Switch3/3, Switch2/3
  Switch3/1 -> Bus Creator1/3  "up"
  Switch2/1 -> Bus Creator1/4  "period"
  Shift Arithmetic1/1 -> Switch3/1
  Abs/1 -> Compare To Constant/1
  Constant3/1 -> Switch2/1, Shift Arithmetic1/1
  Constant5/1 -> Bus Creator1/1  "enable"
  Sign/1 -> Saturation1/1
  Saturation1/1 -> Data Type Conversion/1
  Data Type Conversion/1 -> Bus Creator1/2  "direction"
  rudderAngle/1 -> Add/1

== system code_gen_man_bin/Controller/RC Inputs/Map PWM values to Actuator Signals/Throttle Command ==
  speed : Inport
  Bus Creator : BusCreator
  Compare To Zero : simulink/Logic and Bit Operations/Compare To Zero  SystemSampleTime=-1  relop=~=  LogicOutDataTypeMode=boolean
  Detect Change : simulink/Logic and Bit Operations/Detect Change  SystemSampleTime=-1  vinit=0
  Logical Operator : Logic  AllPortsSameDT=off  OutDataTypeMode=boolean  LogicDataType=fixdt(0, 8)  OutDataTypeStr=boolean
  Mux Everything : Subsystem
  Trigger Events : Subsystem
  command : Outport  OutDataType=sfix(16)  OutScaling=2^0
  wires:
  Bus Creator/1 -> command/1
  speed/1 -> Trigger Events/1(Throttle), Compare To Zero/1, Mux Everything/3(Throttle), Detect Change/1
  Mux Everything/1(iden) -> Bus Creator/1  "identifier"
  Mux Everything/3(size) -> Bus Creator/3  "size"
  Mux Everything/4(trig) -> Bus Creator/4  "trigger"
  Mux Everything/2(data) -> Bus Creator/2  "data"
  Trigger Events/1(Change Speed) -> Mux Everything/1(speed)
  Logical Operator/1 -> Mux Everything/2(enable)
  Compare To Zero/1 -> Logical Operator/1
  Detect Change/1 -> Logical Operator/2

== system code_gen_man_bin/Controller/Radio Control Inputs1/Calibration/Store rudder range to memory ==
  rudderRange : Inport
  Constant : Constant  Value=11  OutDataType=fixdt(1, 16)  OutScaling=2^0  OutDataTypeStr=Inherit: Inherit via back propagation
  Constant1 : Constant  Value=10  OutDataType=fixdt(1, 16)  OutScaling=2^0  OutDataTypeStr=Inherit: Inherit via back propagation
  Demux : Demux  Outputs=2
  Store rudder range  maximum to memory [DEE.c] : dsPICdrivers/OTHERS/C Function Call  Tag=dsPIC_dsPIC_CFunctionCall  FctUpdate=Output Function  fctName='DataEEWrite'  INPUT_SIZE=1  INPUT1=uint16  INPUT2=uint8  INPUT3=--  OUTPUT_SIZE=1  OUTPUT1=--  SampleTime=T_step  InputType=[ 4 2 ]  OutputType=[ ]  FctDeclaration=extern void DataEEWrite(uint16_T u1, uint8_T u2);  FctCall=DataEEWrite(%u1, %u2);  OrderingInOutPopup=None  FctStart=None  FctStart_Name=Init_onlyOnce  FctStart_Declaration=inline extern void Init_onlyOnce();  FctStart_Call=Init_onlyOnce();  FctInit=None  FctInit_Name=Init_Reset  FctInit_Declaration=inline extern void Init_Reset();  FctInit_Call=Init_Reset();  PinDigitalInput=[]  PinDigitalOutput=[]  AnalogueInput=[]
  Store rudder range  minimum to memory [DEE.c] : dsPICdrivers/OTHERS/C Function Call  Tag=dsPIC_dsPIC_CFunctionCall  FctUpdate=Output Function  fctName='DataEEWrite'  INPUT_SIZE=1  INPUT1=uint16  INPUT2=uint8  INPUT3=--  OUTPUT_SIZE=1  OUTPUT1=--  SampleTime=T_step  InputType=[ 4 2 ]  OutputType=[ ]  FctDeclaration=extern void DataEEWrite(uint16_T u1, uint8_T u2);  FctCall=DataEEWrite(%u1, %u2);  OrderingInOutPopup=None  FctStart=None  FctStart_Name=Init_onlyOnce  FctStart_Declaration=inline extern void Init_onlyOnce();  FctStart_Call=Init_onlyOnce();  FctInit=None  FctInit_Name=Init_Reset  FctInit_Declaration=inline extern void Init_Reset();  FctInit_Call=Init_Reset();  PinDigitalInput=[]  PinDigitalOutput=[]  AnalogueInput=[]
  wires:
  Demux/2 -> Store rudder range  maximum to memory [DEE.c]/1
  Demux/1 -> Store rudder range  minimum to memory [DEE.c]/1
  Constant/1 -> Store rudder range  maximum to memory [DEE.c]/2
  Constant1/1 -> Store rudder range  minimum to memory [DEE.c]/2
  rudderRange/1 -> Demux/1

== system code_gen_man_bin/Controller/Radio Control Inputs1/Calibration/Store throttle range to memory ==
  throttleRange : Inport
  Constant : Constant  Value=13  OutDataType=fixdt(1, 16)  OutScaling=2^0  OutDataTypeStr=Inherit: Inherit via back propagation
  Constant1 : Constant  Value=12  OutDataType=fixdt(1, 16)  OutScaling=2^0  OutDataTypeStr=Inherit: Inherit via back propagation
  Demux : Demux  Outputs=2
  Store throttle range  maximum to memory [DEE.c] : dsPICdrivers/OTHERS/C Function Call  Tag=dsPIC_dsPIC_CFunctionCall  FctUpdate=Output Function  fctName='DataEEWrite'  INPUT_SIZE=1  INPUT1=uint16  INPUT2=uint8  INPUT3=--  OUTPUT_SIZE=1  OUTPUT1=--  SampleTime=T_step  InputType=[ 4 2 ]  OutputType=[ ]  FctDeclaration=extern void DataEEWrite(uint16_T u1, uint8_T u2);  FctCall=DataEEWrite(%u1, %u2);  OrderingInOutPopup=None  FctStart=None  FctStart_Name=Init_onlyOnce  FctStart_Declaration=inline extern void Init_onlyOnce();  FctStart_Call=Init_onlyOnce();  FctInit=None  FctInit_Name=Init_Reset  FctInit_Declaration=inline extern void Init_Reset();  FctInit_Call=Init_Reset();  PinDigitalInput=[]  PinDigitalOutput=[]  AnalogueInput=[]
  Store throttle range  minimum to memory [DEE.c] : dsPICdrivers/OTHERS/C Function Call  Tag=dsPIC_dsPIC_CFunctionCall  FctUpdate=Output Function  fctName='DataEEWrite'  INPUT_SIZE=1  INPUT1=uint16  INPUT2=uint8  INPUT3=--  OUTPUT_SIZE=1  OUTPUT1=--  SampleTime=T_step  InputType=[ 4 2 ]  OutputType=[ ]  FctDeclaration=extern void DataEEWrite(uint16_T u1, uint8_T u2);  FctCall=DataEEWrite(%u1, %u2);  OrderingInOutPopup=None  FctStart=None  FctStart_Name=Init_onlyOnce  FctStart_Declaration=inline extern void Init_onlyOnce();  FctStart_Call=Init_onlyOnce();  FctInit=None  FctInit_Name=Init_Reset  FctInit_Declaration=inline extern void Init_Reset();  FctInit_Call=Init_Reset();  PinDigitalInput=[]  PinDigitalOutput=[]  AnalogueInput=[]
  wires:
  Demux/2 -> Store throttle range  maximum to memory [DEE.c]/1
  Demux/1 -> Store throttle range  minimum to memory [DEE.c]/1
  Constant/1 -> Store throttle range  maximum to memory [DEE.c]/2
  Constant1/1 -> Store throttle range  minimum to memory [DEE.c]/2
  throttleRange/1 -> Demux/1

== system code_gen_man_bin/Controller/Radio Control Inputs1/Calibration/Store track range to memory ==
  trackRange : Inport
  Constant : Constant  Value=15  OutDataType=fixdt(1, 16)  OutScaling=2^0  OutDataTypeStr=Inherit: Inherit via back propagation
  Constant1 : Constant  Value=14  OutDataType=fixdt(1, 16)  OutScaling=2^0  OutDataTypeStr=Inherit: Inherit via back propagation
  Demux : Demux  Outputs=2
  Store track range  maximum to memory [DEE.c] : dsPICdrivers/OTHERS/C Function Call  Tag=dsPIC_dsPIC_CFunctionCall  FctUpdate=Output Function  fctName='DataEEWrite'  INPUT_SIZE=1  INPUT1=uint16  INPUT2=uint8  INPUT3=--  OUTPUT_SIZE=1  OUTPUT1=--  SampleTime=T_step  InputType=[ 4 2 ]  OutputType=[ ]  FctDeclaration=extern void DataEEWrite(uint16_T u1, uint8_T u2);  FctCall=DataEEWrite(%u1, %u2);  OrderingInOutPopup=None  FctStart=None  FctStart_Name=Init_onlyOnce  FctStart_Declaration=inline extern void Init_onlyOnce();  FctStart_Call=Init_onlyOnce();  FctInit=None  FctInit_Name=Init_Reset  FctInit_Declaration=inline extern void Init_Reset();  FctInit_Call=Init_Reset();  PinDigitalInput=[]  PinDigitalOutput=[]  AnalogueInput=[]
  Store track range  minimum to memory [DEE.c] : dsPICdrivers/OTHERS/C Function Call  Tag=dsPIC_dsPIC_CFunctionCall  FctUpdate=Output Function  fctName='DataEEWrite'  INPUT_SIZE=1  INPUT1=uint16  INPUT2=uint8  INPUT3=--  OUTPUT_SIZE=1  OUTPUT1=--  SampleTime=T_step  InputType=[ 4 2 ]  OutputType=[ ]  FctDeclaration=extern void DataEEWrite(uint16_T u1, uint8_T u2);  FctCall=DataEEWrite(%u1, %u2);  OrderingInOutPopup=None  FctStart=None  FctStart_Name=Init_onlyOnce  FctStart_Declaration=inline extern void Init_onlyOnce();  FctStart_Call=Init_onlyOnce();  FctInit=None  FctInit_Name=Init_Reset  FctInit_Declaration=inline extern void Init_Reset();  FctInit_Call=Init_Reset();  PinDigitalInput=[]  PinDigitalOutput=[]  AnalogueInput=[]
  wires:
  Demux/2 -> Store track range  maximum to memory [DEE.c]/1
  Demux/1 -> Store track range  minimum to memory [DEE.c]/1
  Constant/1 -> Store track range  maximum to memory [DEE.c]/2
  Constant1/1 -> Store track range  minimum to memory [DEE.c]/2
  trackRange/1 -> Demux/1

== system code_gen_man_bin/Controller/Radio Control Inputs1/Calibration/Update range from input ==
  note: Update lower range limit.
      | The new value is checked against a sane range of 5000-11000
      | to keep values realistic.
  note: Update upper range limit
  limitRange : Inport
  newValue : Inport  Port=2
  If : If  NumInputs=2  IfExpression=u1 < u2 & u1 > 5000 & u1 >= 0
  If Action Subsystem : Subsystem  TreatAsAtomicUnit=on
  If Action Subsystem1 : Subsystem  TreatAsAtomicUnit=on
  If Action Subsystem2 : Subsystem  TreatAsAtomicUnit=on
  If Action Subsystem3 : Subsystem  TreatAsAtomicUnit=on
  If1 : If  NumInputs=2  IfExpression=u1 > u2 & u1 < 11000 & u1 >= 0
  Merge : Merge
  Merge1 : Merge
  Mux : Mux  Inputs=2
  Selector : Selector  InputPortWidth=2  IndexOptions=Index vector (dialog)  Indices=[1]  OutputSizes=1
  Selector1 : Selector  InputPortWidth=2  IndexOptions=Index vector (dialog)  Indices=[2]  OutputSizes=1
  newRange : Outport
  wires:
  Selector/1 -> If/2, If Action Subsystem1/1(In1)
  Selector1/1 -> If Action Subsystem3/1(In1), If1/2
  Mux/1 -> newRange/1
  Merge1/1 -> Mux/2
  Merge/1 -> Mux/1
  If Action Subsystem3/1(Out1) -> Merge1/2
  If Action Subsystem2/1(Out1) -> Merge1/1
  If1/2 -> If Action Subsystem3/Action
  If1/1 -> If Action Subsystem2/Action
  If Action Subsystem1/1(Out1) -> Merge/2
  If Action Subsystem/1(Out1) -> Merge/1
  If/2 -> If Action Subsystem1/Action
  If/1 -> If Action Subsystem/Action
  newValue/1 -> If Action Subsystem/1(In1), If/1, If Action Subsystem2/1(In1), If1/1
  limitRange/1 -> Selector/1, Selector1/1
